simulink model "pll1_org"  (Simulink 10.0)
settings: Solver=ode45  StartTime=0.0  StopTime=tmax  RelTol=1e-3  EnableMultiTasking=on
undefined symbols (not defined in the file): Ci, Cp1, Cp3, f0, fref, Iidn, Iiup, Ipdn, Ipup, Ki, Kp, N, phiref0, phiv0, Rp2, Rp3, td, vi0, vp0, vp10
libraries: simulink x1
settings Model: Creator=OmarAli  LastModifiedBy=bhisma
settings DataIOCC: LimitDataPoints=on
settings DebuggingCC: UnderspecifiedInitializationDetection=Simplified  MergeDetectMultiDrivingBlocksExec=error  SolverPrmCheckMsg=warning
settings GRTTargetCC: GeneratePreprocessorConditionals=Disable all  CombineOutputUpdateFcns=on  GRTInterface=off
settings ConfigComp: CovExternalEMLEnable=off  CovSFcnEnable=off

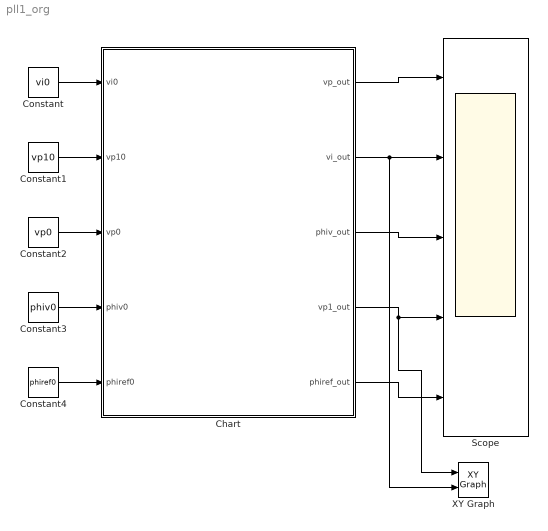
== system pll1_org ==
  Chart : Stateflow chart  TreatAsAtomicUnit=on
  Constant : Constant  Value=vi0
  Constant1 : Constant  Value=vp10
  Constant2 : Constant  Value=vp0
  Constant3 : Constant  Value=phiv0
  Constant4 : Constant  Value=phiref0
  Scope : Scope  NumInputPorts=5
  XY Graph : simulink/Sinks/XY Graph  xmin=-5  xmax=5  ymin=-5  ymax=5  st=-1
  wires:
  Constant/1 -> Chart/1(vi0)
  Constant1/1 -> Chart/2(vp10)
  Constant2/1 -> Chart/3(vp0)
  Constant3/1 -> Chart/4(phiv0)
  Constant4/1 -> Chart/5(phiref0)
  Chart/1(vp_out) -> Scope/1
  Chart/2(vi_out) -> XY Graph/2, Scope/2
  Chart/3(phiv_out) -> Scope/3
  Chart/4(vp1_out) -> XY Graph/1, Scope/4
  Chart/5(phiref_out) -> Scope/5

== stateflow chart Chart ==
  settings: updateMethod=CONTINUOUS
  state both_0
    du:
    vi_dot = 0;
    vp1_dot = -1*( vp1/Cp1)*(1/Rp2 + 1/Rp3) + vp/(Cp1 * Rp3);
    vp_dot = vp1/(Cp3*Rp3) - vp/(Cp3 * Rp3);
    phiv_dot = vi*Ki/N + vp * Kp/N + 2*pi* f0/N;
    phiref_dot = 2*pi*fref;
    t_dot = 1;
    vi_out = vi;
    vp1_out = vp1;
    vp_out = vp;
    phiv_out = phiv;
    phiref_out = phiref;
  state up_1
    du:
    vi_dot = Iiup/Ci;
    vp1_dot = -1*( vp1/Cp1)*(1/Rp2 + 1/Rp3) + vp/(Cp1 * Rp3) + Ipup / Cp1;
    vp_dot = vp1/(Cp3*Rp3) - vp/(Cp3 * Rp3);
    phiv_dot = vi*Ki/N + vp * Kp/N + 2*pi* f0/N;
    phiref_dot = 2*pi*fref;
    t_dot = 1;
    vi_out = vi;
    vp1_out = vp1;
    vp_out = vp;
    phiv_out = phiv;
    phiref_out = phiref;
  state dn_1
    du:
    vi_dot = Iidn/Ci;
    vp1_dot = -1*( vp1/Cp1)*(1/Rp2 + 1/Rp3) + vp/(Cp1 * Rp3) + Ipdn / Cp1;
    vp_dot = vp1/(Cp3*Rp3) - vp/(Cp3 * Rp3);
    phiv_dot = vi*Ki/N + vp * Kp/N + 2*pi* f0/N;
    phiref_dot = 2*pi*fref;
    t_dot = 1;
    vi_out = vi;
    vp1_out = vp1;
    vp_out = vp;
    phiv_out = phiv;
    phiref_out = phiref;
  state both_1
    du:
    vi_dot = (Iiup+Iidn)/Ci;
    vp1_dot = -1*( vp1/Cp1)*(1/Rp2 + 1/Rp3) + vp/(Cp1 * Rp3) + (Ipup+Ipdn) / Cp1;
    vp_dot = vp1/(Cp3*Rp3) - vp/(Cp3 * Rp3);
    phiv_dot = vi*Ki/N + vp * Kp/N + 2*pi* f0/N;
    phiref_dot = 2*pi*fref;
    t_dot = 1;
    vi_out = vi;
    vp1_out = vp1;
    vp_out = vp;
    phiv_out = phiv;
    phiref_out = phiref;
  (default) -> both_0 : {vi = vi0;
      | vp1 = vp10;
      | vp = vp0;
      | phiv = phiv0;
      | phiref = phiref0;}
  both_0 -> up_1 [order 2] : [phiref >= 2*pi]
      | {phiv = phiv - 2*pi;
      | phiref = 0;}
  both_0 -> dn_1 [order 1] : [phiv>= 2*pi]
      | {phiref = phiref - 2*pi;
      | phiv = 0;}
  both_1 -> both_0 : [t >= td]
      | {t = 0;}
  up_1 -> both_1 : [phiv >= 0]
      | {t = 0;}
  dn_1 -> both_1 : [phiref >= 0]
      | {t= 0;}
  data: Cp3 parameter double; Ki parameter double; vi local double; Kp parameter double; vp1 local double; Cp1 parameter double; Rp2 parameter double; Rp3 parameter double; vp local double; f0 parameter double; fref parameter double; Iiup parameter double; Ci parameter double; Ipup parameter double; Ipdn parameter double; Iidn parameter double; td parameter double; vp_out output double; vi_out output double; phiv_out output double; vp1_out output double; phiref_out output double; phiv local double; phiref local double; t local double; N parameter double; vi0 input double; vp10 input double; vp0 input double; phiv0 input double; phiref0 input double
  data vi settings: updateMethod=SF_CONTINUOUS_TIME_DATA
  data vp1 settings: updateMethod=SF_CONTINUOUS_TIME_DATA
  data vp settings: updateMethod=SF_CONTINUOUS_TIME_DATA
  data phiv settings: updateMethod=SF_CONTINUOUS_TIME_DATA
  data phiref settings: updateMethod=SF_CONTINUOUS_TIME_DATA
  data t settings: updateMethod=SF_CONTINUOUS_TIME_DATA
